simulink subsystem "MotoElectricalSystem"  (R2025b)
settings: Solver=VariableStepAuto  StartTime=0.0  StopTime=10.0  RelTol=1e-3
undefined symbols (not defined in the file): PlntDCDCVoltInit
settings Model: Creator=The MathWorks, Inc.  LastModifiedBy=The MathWorks, Inc.
settings RTWCC: GPUComputeCapability=3.5

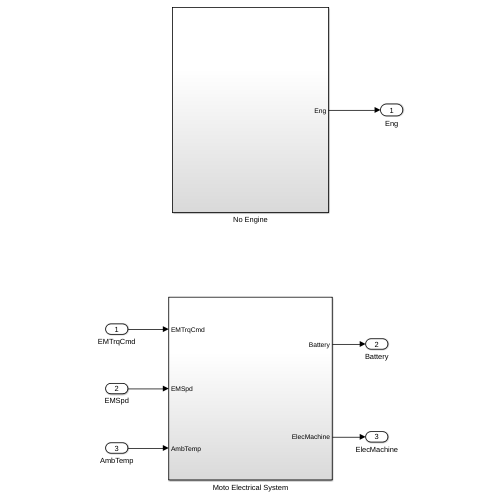
[thumbnail: Simulink's stored preview of the top-level diagram]
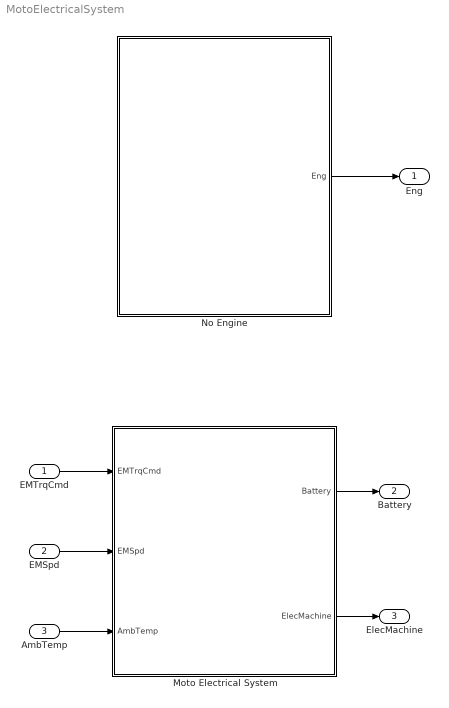
== system MotoElectricalSystem ==
  EMTrqCmd : Inport
  EMSpd : Inport  Port=2
  AmbTemp : Inport  Port=3
  Moto Electrical System : Subsystem  VariantControl=Moto Electrical System 1EM
  No Engine : Subsystem  VariantControl=No Engine
  Eng : Outport
  Battery : Outport  Port=2
  ElecMachine : Outport  Port=3
  wires:
  AmbTemp/1 -> Moto Electrical System/3(AmbTemp)
  EMSpd/1 -> Moto Electrical System/2(EMSpd)
  EMTrqCmd/1 -> Moto Electrical System/1(EMTrqCmd)
  Moto Electrical System/2(ElecMachine) -> ElecMachine/1
  Moto Electrical System/1(Battery) -> Battery/1
  No Engine/1(Eng) -> Eng/1

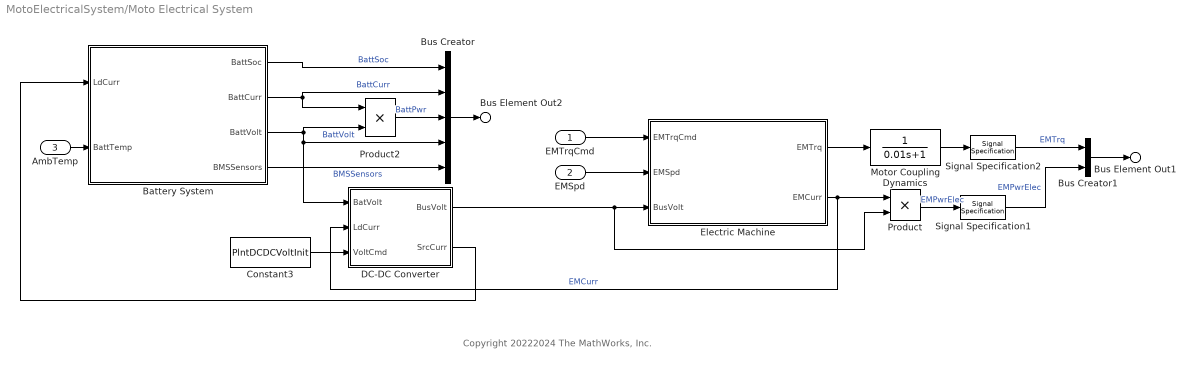
== system MotoElectricalSystem/Moto Electrical System ==
  note: Copyright 20222024 The MathWorks, Inc.
  EMTrqCmd : Inport
  EMSpd : Inport  Port=2
  AmbTemp : Inport  Port=3
  Battery System : Subsystem  Variant=on  VariantControlMode=label  LabelModeActiveChoice=Ideal Voltage Source
  Bus Creator : BusCreator  Inputs=5
  Bus Creator1 : BusCreator  Inputs=2
  Constant3 : Constant  Value=PlntDCDCVoltInit  SampleTime=-1
  DC-DC Converter : Subsystem  Variant=on  VariantControlMode=label  VariantControl=Choice  LabelModeActiveChoice=No DC-DC Converter
  Electric Machine : Subsystem  Variant=on  VariantControlMode=label  LabelModeActiveChoice=Mapped EM
  Motor Coupling Dynamics : TransferFcn  Denominator=[0.01 1]
  Product : Product
  Product2 : Product
  Signal Specification1 : SignalSpecification  Unit=W
  Signal Specification2 : SignalSpecification  Unit=N*m
  Bus Element Out2 : Outport  PortName=Battery
  Bus Element Out1 : Outport  Port=2  PortName=ElecMachine
  wires:
  Product/1 -> Signal Specification1/1  "EMPwrElec"
  Motor Coupling Dynamics/1 -> Signal Specification2/1
  AmbTemp/1 -> Battery System/2(BattTemp)
  Battery System/2(BattCurr) -> Bus Creator/2, Product2/1  "BattCurr"
  EMTrqCmd/1 -> Electric Machine/1(EMTrqCmd)
  Electric Machine/2(EMCurr) -> DC-DC Converter/2(LdCurr), Product/1  "EMCurr"
  Battery System/1(BattSoc) -> Bus Creator/1  "BattSoc"
  EMSpd/1 -> Electric Machine/2(EMSpd)
  Battery System/3(BattVolt) -> DC-DC Converter/1(BatVolt), Bus Creator/4, Product2/2  "BattVolt"
  Product2/1 -> Bus Creator/3  "BattPwr"
  Signal Specification1/1 -> Bus Creator1/2  "EMPwrElec"
  Bus Creator1/1 -> Bus Element Out1/1
  Signal Specification2/1 -> Bus Creator1/1  "EMTrq"
  Electric Machine/1(EMTrq) -> Motor Coupling Dynamics/1
  Bus Creator/1 -> Bus Element Out2/1
  DC-DC Converter/1(BusVolt) -> Product/2, Electric Machine/3(BusVolt)
  DC-DC Converter/2(SrcCurr) -> Battery System/1(LdCurr)
  Constant3/1 -> DC-DC Converter/3(VoltCmd)
  Battery System/4(BMSSensors) -> Bus Creator/5  "BMSSensors"

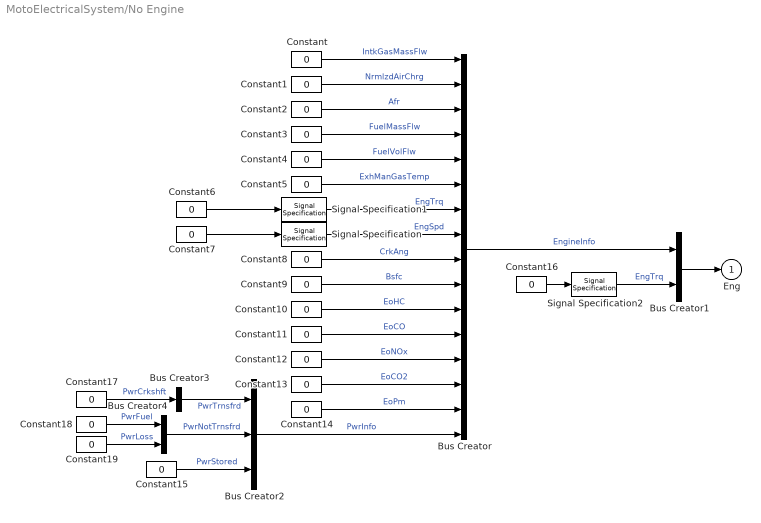
== system MotoElectricalSystem/No Engine ==
  Bus Creator : BusCreator  Inputs=16
  Bus Creator1 : BusCreator  Inputs=2
  Bus Creator2 : BusCreator  Inputs=3
  Bus Creator3 : BusCreator  Inputs=1
  Bus Creator4 : BusCreator  Inputs=2
  Constant{,1..19} (20 alike) : Constant  Value=0
  Signal Specification : SignalSpecification  Unit=rpm
  Signal Specification1 : SignalSpecification  Unit=N*m
  Signal Specification2 : SignalSpecification  Unit=N*m
  Eng : Outport
  wires:
  Constant16/1 -> Signal Specification2/1
  Constant6/1 -> Signal Specification1/1
  Constant7/1 -> Signal Specification/1
  Constant19/1 -> Bus Creator4/2  "PwrLoss"
  Constant18/1 -> Bus Creator4/1  "PwrFuel"
  Constant17/1 -> Bus Creator3/1  "PwrCrkshft"
  Constant15/1 -> Bus Creator2/3  "PwrStored"
  Bus Creator4/1 -> Bus Creator2/2  "PwrNotTrnsfrd"
  Bus Creator3/1 -> Bus Creator2/1  "PwrTrnsfrd"
  Signal Specification2/1 -> Bus Creator1/2  "EngTrq"
  Bus Creator/1 -> Bus Creator1/1  "EngineInfo"
  Bus Creator1/1 -> Eng/1
  Constant5/1 -> Bus Creator/6  "ExhManGasTemp"
  Constant/1 -> Bus Creator/1  "IntkGasMassFlw"
  Constant12/1 -> Bus Creator/13  "EoNOx"
  Constant13/1 -> Bus Creator/14  "EoCO2"
  Bus Creator2/1 -> Bus Creator/16  "PwrInfo"
  Constant3/1 -> Bus Creator/4  "FuelMassFlw"
  Constant1/1 -> Bus Creator/2  "NrmlzdAirChrg"
  Constant14/1 -> Bus Creator/15  "EoPm"
  Constant11/1 -> Bus Creator/12  "EoCO"
  Constant10/1 -> Bus Creator/11  "EoHC"
  Constant8/1 -> Bus Creator/9  "CrkAng"
  Signal Specification/1 -> Bus Creator/8  "EngSpd"
  Constant4/1 -> Bus Creator/5  "FuelVolFlw"
  Signal Specification1/1 -> Bus Creator/7  "EngTrq"
  Constant2/1 -> Bus Creator/3  "Afr"
  Constant9/1 -> Bus Creator/10  "Bsfc"

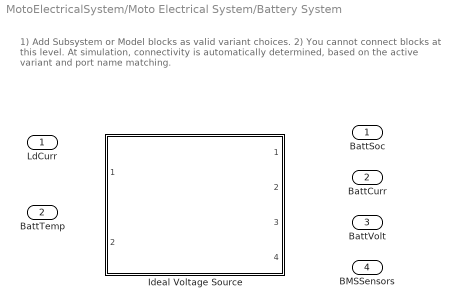
== system MotoElectricalSystem/Moto Electrical System/Battery System ==
  note: 1) Add Subsystem or Model blocks as valid variant choices.
      | 2) You cannot connect blocks at this level. At simulation, connectivity is automatically
      | determined, based on the active variant and port name matching.
  LdCurr : Inport
  BattTemp : Inport  Port=2
  Ideal Voltage Source : Subsystem  VariantControl=Ideal Voltage Source  ReferencedSubsystem=IdealVoltageSource
  BattSoc : Outport  VectorParamsAs1DForOutWhenUnconnected=off
  BattCurr : Outport  Port=2  VectorParamsAs1DForOutWhenUnconnected=off
  BattVolt : Outport  Port=3  VectorParamsAs1DForOutWhenUnconnected=off
  BMSSensors : Outport  Port=4  VectorParamsAs1DForOutWhenUnconnected=off

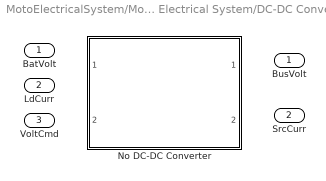
== system MotoElectricalSystem/Moto Electrical System/DC-DC Converter ==
  BatVolt : Inport
  LdCurr : Inport  Port=2
  VoltCmd : Inport  Port=3
  No DC-DC Converter : Subsystem  VariantControl=No DC-DC Converter  ReferencedSubsystem=NoDCDCConverter
  BusVolt : Outport
  SrcCurr : Outport  Port=2

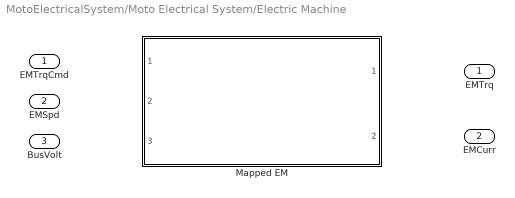
== system MotoElectricalSystem/Moto Electrical System/Electric Machine ==
  EMTrqCmd : Inport
  EMSpd : Inport  Port=2
  BusVolt : Inport  Port=3
  Mapped EM : Subsystem  VariantControl=Mapped EM  ReferencedSubsystem=ElectricMachine1
  EMTrq : Outport  VectorParamsAs1DForOutWhenUnconnected=off
  EMCurr : Outport  Port=2  VectorParamsAs1DForOutWhenUnconnected=off
